simulink model "SPERTE_printer_RC"  (R2024b)
settings: Solver=FixedStepDiscrete  StartTime=0.0  StopTime=tsim  FixedStep=Ts  RelTol=1e-3  EnableMultiTasking=on
InitFcn:
  | Fs = 1000; Ts = 1/Fs;tsim = Inf;
values from neighbouring files (symbols this model uses):
  N = length(r)    [SimExpRC_SPERTE.m]
  N_RC_activate = 5    [SimExpRC_SPERTE.m]
  N_trial = 50    [SimExpRC_SPERTE.m]
  p_Q = M    (= 50)    [DesignControllerRC.m]
undefined symbols (not defined in the file or in its folder): DiscIntNeverNeededParam, p_L
libraries: simulink x7, sperte_lib x3, cstblocks x2
(part 1 of 2)
settings Model: SimulationMode=external  ExtModeTrigDuration=2  Creator=glife  LastModifiedBy=20202036
settings SolverCC: AlgebraicLoopSolver=TrustRegion  PositivePriorityOrder=on
settings DataIOCC: SaveOutput=off  DSMLogging=off  SaveTime=off  ReturnWorkspaceOutputs=off
settings OptimizationCC: EnhancedBackFolding=on  PassReuseOutputArgsThreshold=0  MaxStackSize=200000  OptimizeBlockOrder=speed  DifferentSizesBufferReuse=on  OptimizationCustomize=off
settings DebuggingCC: ParameterTunabilityLossMsg=error  UnconnectedInputMsg=warning  UnconnectedOutputMsg=warning  UnconnectedLineMsg=warning  ArithmeticOperatorsInVariantConditions=warning
settings HardwareCC: ProdBitPerLong=64  ProdLargestAtomicInteger=LongLong  ProdLargestAtomicFloat=Double  ProdLongLongMode=on  ProdHWDeviceType=ARM Compatible->ARM Cortex-A (64-bit)  UseEmbeddedCoderFeatures=off
settings ModelReferenceCC: EnableRefExpFcnMdlSchedulingChecks=on
settings SFSimCC: CustomCodeUndefinedFunction=UseInterfaceOnly
settings RTWCC: Description=Embedded Coder  SystemTargetFile=ert.tlc  HardwareBoard=Raspberry Pi (64bit)  TLCOptions="-aInlineSetEventsForThisBaseRateFcn=TLC_FALSE -aSuppressMultiTaskScheduler=TLC_FALSE  -aRateBasedStepFcn=0"  TemplateMakefile=ert_default_tmf  PostCodeGenCommand=codertarget.postCodeGenHookCommand(h); SPERTE_postGenFunc(modelName, buildInfo);  CustomSource=MW_custom_RTOS.c  CustomDefine=COREAFFINITYREQUIRED  Toolchain=GNU GCC Embedded Linux  BuildConfiguration=Faster Runs  GPUComputeCapability=3.5
settings CodeAppCC: ForceParamTrailComments=on  OperatorAnnotations=on
settings ERTTargetCC: CodeReplacementLibrary=GNU C99 extensions  ERTCustomFileBanners=off  SupportContinuousTime=on  SupportNonInlinedSFcns=on  RemoveResetFunc=off  SupportVariableSizeSignals=on  ModelStepFunctionPrototypeControlCompliant=off  ExtMode=on  ExtModeTransport=2  ExtModeStaticAlloc=on  ExtModeMexFile=ext_xcp  ExtModeMexArgs='131.155.56.35' 1 17725  ExtModeIntrfLevel=Level2 - Open  InlinedParameterPlacement=Hierarchical  ERTSrcFileBannerTemplate=codertarget_code_template.cgt  ERTHdrFileBannerTemplate=codertarget_code_template.cgt  ERTDataSrcFileTemplate=codertarget_code_template.cgt  ERTDataHdrFileTemplate=codertarget_code_template.cgt  DynamicArrayContainerType=coder::array

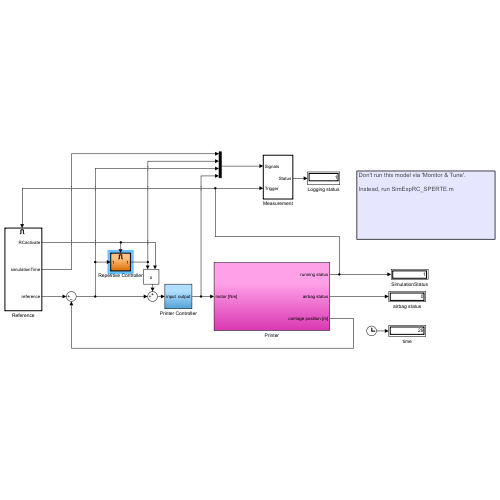
[thumbnail: Simulink's stored preview of the top-level diagram]
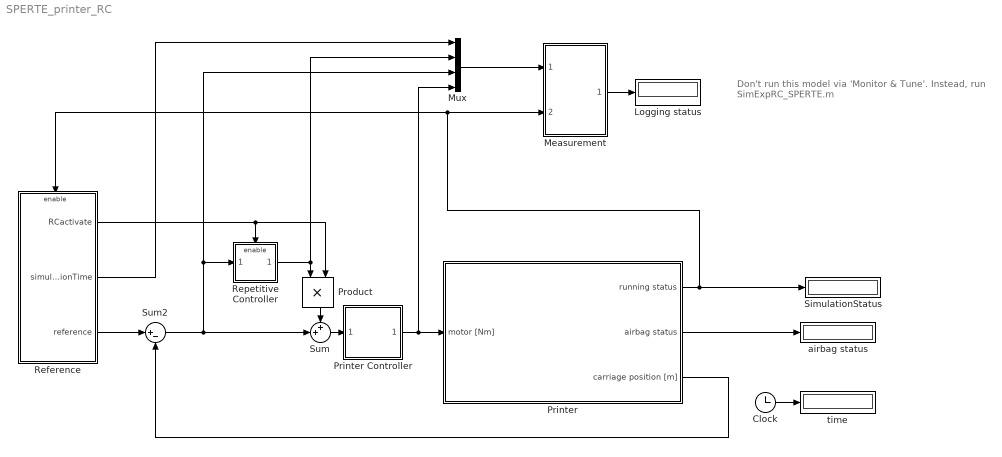
== system SPERTE_printer_RC ==
  note: Don't run this model via 'Monitor & Tune'.
      |
      | Instead, run SimExpRC_SPERTE.m
  Clock : Clock
  Logging status : Display
  Measurement : Subsystem  TreatAsAtomicUnit=on
  Mux : Mux
  Printer : Subsystem
  Printer Controller : Subsystem
  Product : Product
  Reference : Subsystem  TreatAsAtomicUnit=on
  Repetitive Controller : Subsystem  InitFcn=load('RCController.mat');
  SimulationStatus : Display
      settings: Decimation=50
  Sum : Sum  Inputs=++|
  Sum2 : Sum  Inputs=|+-
  airbag status : Display
      settings: Decimation=50
  time : Display
      settings: Decimation=50
  wires:
  Printer/3(carriage position [m]) -> Sum2/2
  Printer/2(airbag status) -> airbag status/1
  Sum2/1 -> Mux/3, Repetitive Controller/1(Input), Sum/2
  Printer Controller/1(output) -> Mux/4, Printer/1(motor [Nm])
  Clock/1 -> time/1
  Reference/3(reference) -> Sum2/1
  Mux/1 -> Measurement/1(Signals)
  Measurement/1(Status) -> Logging status/1
  Sum/1 -> Printer Controller/1(input)
  Product/1 -> Sum/1
  Repetitive Controller/1(Output) -> Mux/2, Product/1
  Reference/1(RCactivate) -> Product/2, Repetitive Controller/Enable
  Reference/2(simulationTime) -> Mux/1
  Printer/1(running status) -> Measurement/2(Trigger), Reference/Enable, SimulationStatus/1

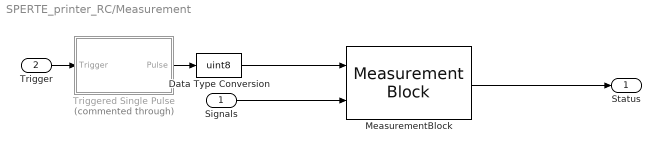
== system SPERTE_printer_RC/Measurement ==
  Signals : Inport
  Trigger : Inport  Port=2
  Data Type Conversion : DataTypeConversion  OutDataTypeStr=uint8  SaturateOnIntegerOverflow=off  RndMeth=Floor
  MeasurementBlock : sperte_lib/Measurement/Measurement Block  Description=|  Priority=-1  N_samples=N*N_trial  triggertype=0  trigger_command=1
      | Perform on-demand measurements to file using this block.
      | 
      | It can be used in 2 ways:
      | 1) Set the mask triggertype parameter to manual and use the trigger input signal to trigger a measurement.
      | You can do this by providing a 0 to 1 transition.
      | Keep it low after you start/complete the measurement, or it will measure again.
      | A file is created with measurement_0,1,2... etc
      | 
      | 2) Keep the model running, and trigger a measurement from the commandline or Matlab script.
      | For example:
      | 
      | % How many samples to measure?
      | N_samples = Fs*5;
      | % Do the measurement
      | SPERTE_Perform_Measurement(N_samples);
      | % Get the latest file
      | file_list = SPERTE_Get_Latest_Measurement(p,1,'./data');
      | % How many signals did you record?
      | N_signals = 3;
      | % Convert the .bin to .mat and return the results
      | measurement = SPERTE_Bin_To_Mat(file_list,N_signals);
      settings: SourceProductName=SPERTE library
  Triggered Single Pulse : Subsystem  Commented=through  TreatAsAtomicUnit=on  mask(single pulse generation){p_wid=20}
      mask prompts: p_wid "pulse width (number of samples)"
      mask help: This block generate a single pulse whenever a trigger happen. The pulse width must specified as a number of samples. for example if your sampling time is 0.1s and you want 3s pulse , then you should enter 30 as a pulse width.
      mask Display:
      | plot([0],[0])
      | plot([11],[0])
      | plot([5],[0.5])
      | plot([4 5 5 6 6 7],[0 0 0.25 0.25 0 0])
      | plot([5],[-0.3])
      | 
      | port_label('output', 1, 'Pulse')
      | port_label('input', 1, 'Trigger')
  Status : Outport
  wires:
  Data Type Conversion/1 -> MeasurementBlock/1
  MeasurementBlock/1 -> Status/1
  Signals/1 -> MeasurementBlock/2
  Triggered Single Pulse/1(Pulse) -> Data Type Conversion/1
  Trigger/1 -> Triggered Single Pulse/1(Trigger)

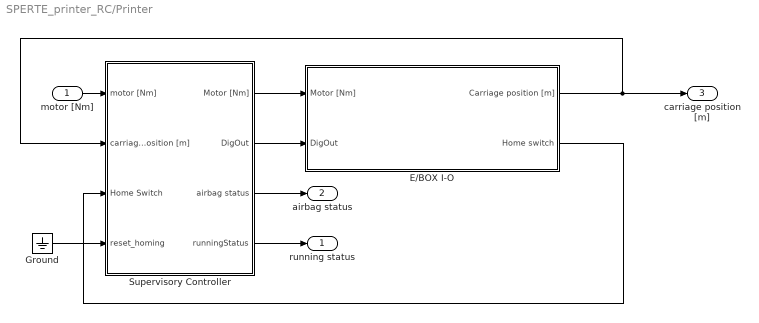
== system SPERTE_printer_RC/Printer ==
  motor [Nm] : Inport
  E/BOX I-O : Subsystem
  Ground : Ground
  Supervisory Controller : Subsystem
  running status : Outport
  airbag status : Outport  Port=2
  carriage position [m] : Outport  Port=3
  wires:
  E/BOX I-O/1(Carriage position [m]) -> Supervisory Controller/2(carriage position [m]), carriage position [m]/1
  Supervisory Controller/1(Motor [Nm]) -> E/BOX I-O/1(Motor [Nm])
  E/BOX I-O/2(Home switch) -> Supervisory Controller/3(Home Switch)
  motor [Nm]/1 -> Supervisory Controller/1(motor [Nm])
  Supervisory Controller/3(airbag status) -> airbag status/1
  Supervisory Controller/4(runningStatus) -> running status/1
  Supervisory Controller/2(DigOut) -> E/BOX I-O/2(DigOut)
  Ground/1 -> Supervisory Controller/4(reset_homing)

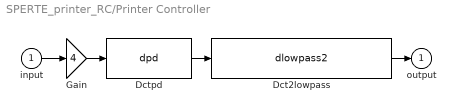
== system SPERTE_printer_RC/Printer Controller ==
  input : Inport
  Dct2lowpass : S-Function  FunctionName=dlowpass2  Parameters=f_den, b_den, 0.001  SFunctionDeploymentMode=off  EnableBusSupport=off  mask(dctools){f_den=40, b_den=0.7}
      mask prompts: f_den "Pole [Hz]"; b_den "Damping pole [-]"
      mask help: This block implements a discrete time 2nd order lowpass filter.
      mask Display: disp('DCT 2nd order lowpass')
  Dctpd : S-Function  FunctionName=dpd  Parameters=kp, kv, 0.001  SFunctionDeploymentMode=off  EnableBusSupport=off  mask(dctools){kp=40, kv=1}
      mask help: This block implements a discrete time pd filter.
      mask Display: disp('DCT pd')
  Gain : Gain  Gain=4  SaturateOnIntegerOverflow=on  OutDataTypeStr=Inherit: Same as input  ParamDataTypeStr=Inherit: Same as input
  output : Outport
  wires:
  input/1 -> Gain/1
  Gain/1 -> Dctpd/1
  Dctpd/1 -> Dct2lowpass/1
  Dct2lowpass/1 -> output/1

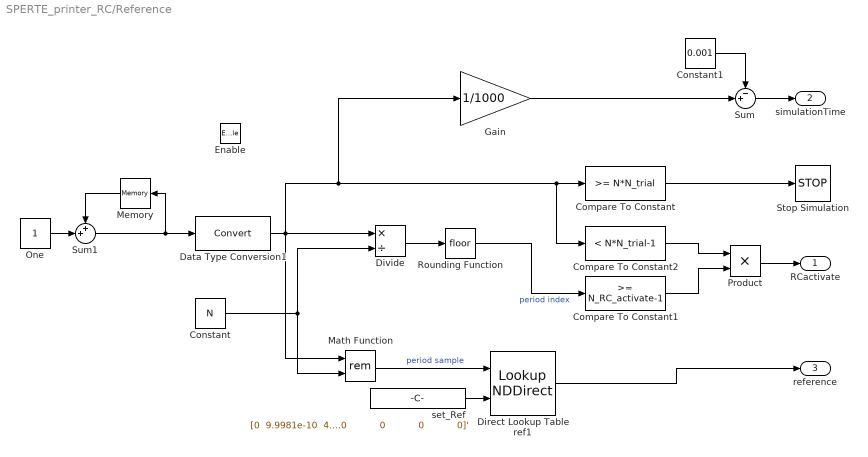
== system SPERTE_printer_RC/Reference ==
  Enable : EnablePort  StatesWhenEnabling=reset
  Compare To Constant : simulink/Logic and Bit Operations/Compare To Constant  relop=>=  const=N*N_trial  OutDataTypeStr=boolean
  Compare To Constant1 : simulink/Logic and Bit Operations/Compare To Constant  relop=>=  const=N_RC_activate-1  OutDataTypeStr=boolean
  Compare To Constant2 : simulink/Logic and Bit Operations/Compare To Constant  relop=<  const=N*N_trial-1  OutDataTypeStr=boolean
  Constant : Constant  Value=N
  Constant1 : Constant  Value=0.001
  Data Type Conversion1 : DataTypeConversion  SaturateOnIntegerOverflow=off  RndMeth=Floor
  Direct Lookup Table ref1 : LookupNDDirect  NumberOfTableDimensions=1  TableIsInput=on  Table=[4 5 ;16 19 ]  DiagnosticForOutOfRangeInput=Error
  Divide : Product  Inputs=*/
  Gain : Gain  Gain=1/1000
  Math Function : Math  Operator=rem  SignedPower=on
  Memory : Memory
  One : Constant  OutDataTypeStr=Inherit: Inherit via back propagation
  Product : Product
  Rounding Function : Rounding
  Stop Simulation : Stop
  Sum : Sum  Inputs=-+|
  Sum1 : Sum  Inputs=++|
  set_Ref : Constant  Value="[0  9.9981e-10  4.9991e-09  1.4997e-08  3.4993e-08  6.9987e-08  1.2598e-07  2.0996e-07  3.2994e-07  4.9491e-07  7.1487e-07  1.0008e-06  1.3647e-06  1.8197e-06  2.3796e-06  3.0594e-06  3.8753e-06  4.8441e-06  5.9839e-06  7.3136e-06  8.8533e-06  1.0624e-05  1.2648e-05  1.4947e-05  1.7547e-05  2.0471e-05  2.3747e-05    2.74e-05  3.1459e-05  3.5953e-05  4.0912e-05  4.6367e-05   5.235e-05  5.8894e-05  6.6033e-05  7.3801e-05  8.2236e-05  9.1373e-05  0.00010125  0.00011191  0.00012339  0.00013573  0.00014897  0.00016315  0.00017833  0.00019454  0.00021184  0.00023026  0.00024985  0.00027067  0.00029277  0.00031619  0.00034099  0.00036722  0.00039494  0.00042419  0.00045504  0.00048754  0.00052176  0.00055774  0.00059555  0.00063526  0.00067691  0.00072058  0.00076633  0.00081422  0.00086431  0.00091665  0.00097131   0.0010283   0.0010878   0.0011497   0.0012142   0.0012813    0.001351   0.0014234   0.0014986   0.0015765   0.0016573    0.001741   0.0018276   0.0019172   0.0020098   0.0021054   0.0022042   0.0023062   0.0024113   0.0025196   0.0026312   0.0027461   0.0028644    0.002986    0.003111   0.0032395   0.0033715   0.0035069   0.0036459   0.0037884   0.0039346   0.0040843   0.0042377   0.0043948   0.0045555     0.00472   0.0048882   0.0050602   0.0052359   0.0054154   0.0055988    0.005786    0.005977   0.0061719   0.0063707   0.0065734   0.0067799   0.0069904   0.0072048   0.0074232   0.0076454   0.0078717   0.0081018    0.008336   0.0085741   0.0088161   0.0090622   0.0093122   0.0095661   0.0098241    0.010086    0.010352    0.010622    0.010895    0.011173    0.011455     0.01174     0.01203    0.012323    0.012621    0.012922    0.013227    0.013536    0.013849    0.014165    0.014486     0.01481    0.015138     0.01547    0.015806    0.016145    0.016488    0.016834    0.017185    0.017538    0.017896    0.018257    0.018621     0.01899    0.019361    0.019736    0.020114    0.020496    0.020881     0.02127    0.021661    0.022056    0.022454    0.022855     0.02326    0.023667    0.024078    0.024491    0.024907    0.025327    0.025749    0.026173    0.026601    0.027031    0.027464      0.0279    0.028338    0.028778    0.029221    0.029667    0.030114    0.030564    0.031016    0.031471    0.031927    0.032385    0.032846    0.033308    0.033772    0.034238    0.034705    0.035174    0.035645    0.036117    0.036591    0.037066    0.037543    0.038021      0.0385     0.03898    0.039462    0.039945    0.040428    0.040913    0.041399    0.041886    0.042373    0.042862    0.043351    0.043841    0.044332    0.044824    0.045316    0.045809    0.046302    0.046796    0.047291    0.047786    0.048281    0.048777    0.049274     0.04977    0.050268    0.050765    0.051263    0.051761    0.052259    0.052757    0.053256    0.053755    0.054254    0.054753    0.055252    0.055752    0.056251    0.056751    0.057251     0.05775     0.05825     0.05875     0.05925     0.05975     0.06025     0.06075     0.06125     0.06175     0.06225     0.06275     0.06325     0.06375     0.06425     0.06475     0.06525     0.06575     0.06625     0.06675     0.06725     0.06775     0.06825     0.06875     0.06925     0.06975     0.07025     0.07075     0.07125     0.07175     0.07225     0.07275     0.07325     0.07375     0.07425     0.07475     0.07525     0.07575     0.07625     0.07675     0.07725     0.07775     0.07825     0.07875     0.07925     0.07975     0.08025     0.08075     0.08125     0.08175     0.08225     0.08275     0.08325     0.08375     0.08425     0.08475     0.08525     0.08575     0.08625     0.08675     0.08725     0.08775     0.08825     0.08875     0.08925     0.08975     0.09025     0.09075     0.09125     0.09175     0.09225     0.09275     0.09325     0.09375     0.09425     0.09475     0.09525     0.09575     0.09625     0.09675     0.09725     0.09775     0.09825     0.09875     0.09925     0.09975     0.10025     0.10075     0.10125     0.10175     0.10225     0.10275     0.10325     0.10375     0.10425 ...(+17687 chars)]'"
  RCactivate : Outport  InitialOutput=0
  simulationTime : Outport  Port=2  InitialOutput=0
  reference : Outport  Port=3  InitialOutput=0
  wires:
  Divide/1 -> Rounding Function/1
  Rounding Function/1 -> Compare To Constant1/1  "period index"
  Compare To Constant2/1 -> Product/1
  Data Type Conversion1/1 -> Divide/1, Gain/1, Compare To Constant2/1, Compare To Constant/1, Math Function/1
  Compare To Constant/1 -> Stop Simulation/1
  Direct Lookup Table ref1/1 -> reference/1
  Gain/1 -> Sum/2
  Constant/1 -> Divide/2, Math Function/2
  Product/1 -> RCactivate/1
  Sum1/1 -> Data Type Conversion1/1, Memory/1
  Compare To Constant1/1 -> Product/2
  Math Function/1 -> Direct Lookup Table ref1/1  "period sample"
  set_Ref/1 -> Direct Lookup Table ref1/2
  Memory/1 -> Sum1/1
  One/1 -> Sum1/2
  Sum/1 -> simulationTime/1
  Constant1/1 -> Sum/1

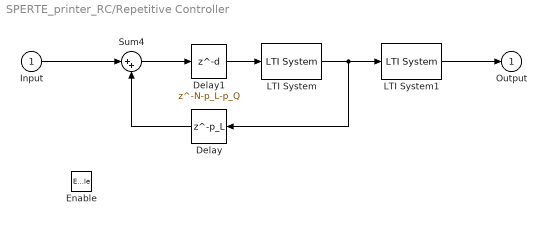
== system SPERTE_printer_RC/Repetitive Controller ==
  Input : Inport
  Enable : EnablePort  StatesWhenEnabling=reset
  Delay : Delay  DelayLength=p_L  InitialCondition=0
  Delay1 : Delay  DelayLength=N-p_L-p_Q  InitialCondition=0
  LTI System : cstblocks/LTI System  sys=Q_c  IC=[]  PadeOrder=0
  LTI System1 : cstblocks/LTI System  sys=L_c  IC=[]  PadeOrder=0
  Sum4 : Sum  Inputs=|++  InputSameDT=on  SaturateOnIntegerOverflow=on  OutDataTypeStr=Inherit: Same as first input
  Output : Outport  InitialOutput=[0]
  wires:
  Input/1 -> Sum4/1
  LTI System1/1 -> Output/1
  Sum4/1 -> Delay1/1
  Delay/1 -> Sum4/2
  Delay1/1 -> LTI System/1
  LTI System/1 -> LTI System1/1, Delay/1

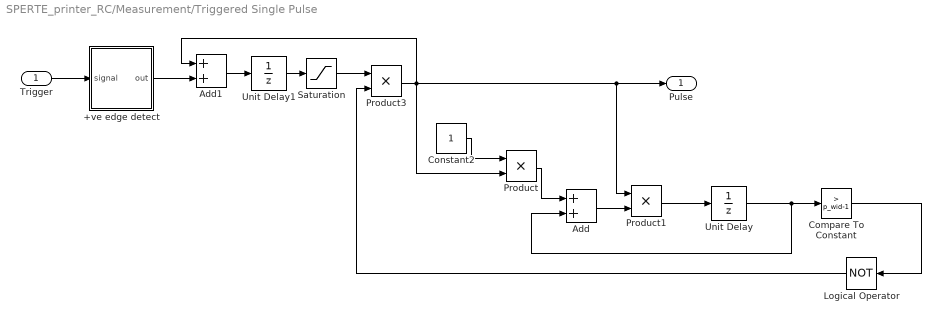
== system SPERTE_printer_RC/Measurement/Triggered Single Pulse ==
  Trigger : Inport
  +ve edge detect : Subsystem
  Add : Sum
  Add1 : Sum
  Compare To Constant : simulink/Logic and Bit Operations/Compare To Constant  relop=>  const=p_wid-1  OutDataTypeStr=boolean
  Constant2 : Constant
  Logical Operator : Logic  Operator=NOT  AllPortsSameDT=off  OutDataTypeStr=boolean
  Product : Product  RndMeth=Zero
  Product1 : Product  RndMeth=Zero
  Product3 : Product  RndMeth=Zero
  Saturation : Saturate  UpperLimit=1  LowerLimit=0
  Unit Delay : UnitDelay  SampleTime=-1  HasFrameUpgradeWarning=on
  Unit Delay1 : UnitDelay  SampleTime=-1  HasFrameUpgradeWarning=on
  Pulse : Outport
  wires:
  Compare To Constant/1 -> Logical Operator/1
  Constant2/1 -> Product/1
  Product/1 -> Add/1
  Unit Delay/1 -> Add/2, Compare To Constant/1
  Trigger/1 -> +ve edge detect/1(signal)
  +ve edge detect/1(out) -> Add1/2
  Add/1 -> Product1/2
  Product1/1 -> Unit Delay/1
  Add1/1 -> Unit Delay1/1
  Unit Delay1/1 -> Saturation/1
  Saturation/1 -> Product3/1
  Product3/1 -> Add1/1, Product/2, Product1/1, Pulse/1
  Logical Operator/1 -> Product3/2

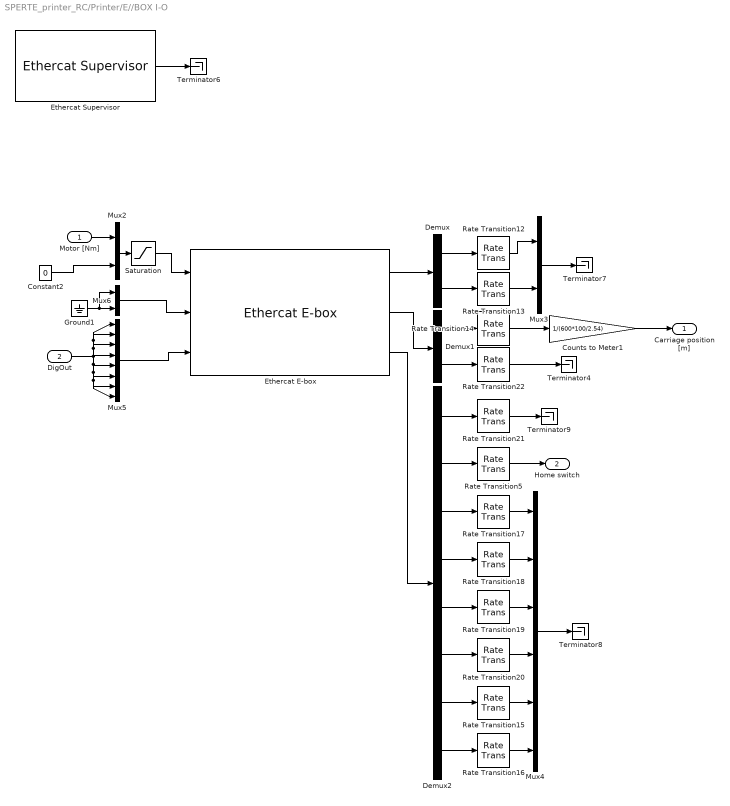
== system SPERTE_printer_RC/Printer/E//BOX I-O ==
  Motor [Nm] : Inport
  DigOut : Inport  Port=2
  Constant2 : Constant  Value=0
  Counts to Meter1 : Gain  Gain=1/(600*100/2.54)
  Demux : Demux  Outputs=2
  Demux1 : Demux  Outputs=2
  Demux2 : Demux  Outputs=8
  Ethercat E-box : sperte_lib/EtherCAT/Ethercat E-box  Priority=-2  link_id=0
      settings: SourceProductName=SPERTE library
  Ethercat Supervisor : sperte_lib/EtherCAT/Ethercat Supervisor  Description=Must be executed first, keep at -1 priority (highest)  Priority=-3  portid=0  ectimeout=500
      settings: SourceProductName=SPERTE library
  Ground1 : Ground
  Mux2 : Mux  Inputs=2
  Mux3 : Mux  Inputs=2
  Mux4 : Mux  Inputs=6
  Mux5 : Mux  Inputs=8
  Mux6 : Mux  Inputs=2
  Rate Transition{5,12..22} (12 alike) : RateTransition
  Saturation : Saturate  UpperLimit=2.5  LowerLimit=-2.5
  Terminator{4,6..9} (5 alike) : Terminator
  Carriage position [m] : Outport
  Home switch : Outport  Port=2
  wires:
  Motor [Nm]/1 -> Mux2/1
  Demux2/2 -> Rate Transition5/1
  Rate Transition5/1 -> Home switch/1
  Saturation/1 -> Ethercat E-box/1
  Ethercat E-box/3 -> Demux2/1
  Ground1/1 -> Mux6/1, Mux6/2
  Ethercat Supervisor/1 -> Terminator6/1
  Ethercat E-box/2 -> Demux1/1
  Constant2/1 -> Mux2/2
  Mux2/1 -> Saturation/1
  Counts to Meter1/1 -> Carriage position [m]/1
  Ethercat E-box/1 -> Demux/1
  Demux/1 -> Rate Transition12/1
  Demux/2 -> Rate Transition13/1
  Rate Transition13/1 -> Mux3/2
  Mux3/1 -> Terminator7/1
  Rate Transition12/1 -> Mux3/1
  Rate Transition14/1 -> Counts to Meter1/1
  Demux1/1 -> Rate Transition14/1
  Demux1/2 -> Rate Transition22/1
  Rate Transition19/1 -> Mux4/3
  Rate Transition18/1 -> Mux4/2
  Rate Transition20/1 -> Mux4/4
  Demux2/8 -> Rate Transition16/1
  Rate Transition17/1 -> Mux4/1
  Demux2/5 -> Rate Transition19/1
  Demux2/6 -> Rate Transition20/1
  Demux2/4 -> Rate Transition18/1
  Rate Transition15/1 -> Mux4/5
  Mux4/1 -> Terminator8/1
  Demux2/3 -> Rate Transition17/1
  Demux2/7 -> Rate Transition15/1
  Rate Transition16/1 -> Mux4/6
  Rate Transition21/1 -> Terminator9/1
  Demux2/1 -> Rate Transition21/1
  Mux5/1 -> Ethercat E-box/3
  DigOut/1 -> Mux5/8, Mux5/7, Mux5/6, Mux5/5, Mux5/4, Mux5/1, Mux5/2, Mux5/3
  Mux6/1 -> Ethercat E-box/2
  Rate Transition22/1 -> Terminator4/1

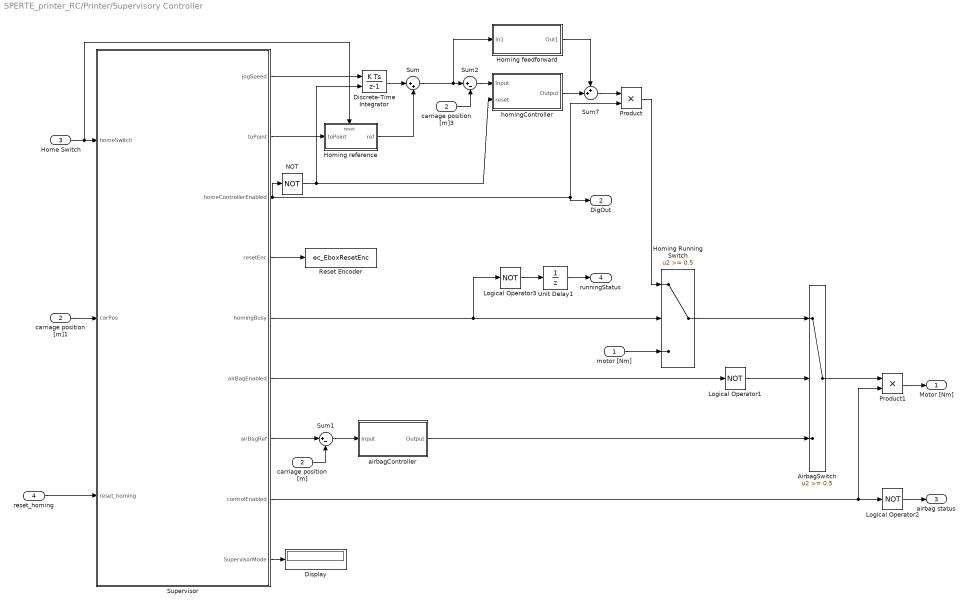
== system SPERTE_printer_RC/Printer/Supervisory Controller ==
  motor [Nm] : Inport
  carriage position [m] : Inport  Port=2
  Home Switch : Inport  Port=3
  reset_homing : Inport  Port=4
  AirbagSwitch : Switch  Threshold=0.5  SaturateOnIntegerOverflow=off  InputSameDT=off
  Discrete-Time Integrator : DiscreteIntegrator  ExternalReset=level  SampleTime=-1  ICPrevOutput=DiscIntNeverNeededParam  ICPrevScaledInput=DiscIntNeverNeededParam
  Display : Display
  Homing Running Switch : Switch  Threshold=0.5  SaturateOnIntegerOverflow=off  InputSameDT=off
  Homing feedforward : Subsystem
  Homing reference : Subsystem
  Logical Operator1 : Logic  Operator=NOT  AllPortsSameDT=off  OutDataTypeStr=boolean
  Logical Operator2 : Logic  Operator=NOT  AllPortsSameDT=off  OutDataTypeStr=boolean
  Logical Operator3 : Logic  Operator=NOT  AllPortsSameDT=off  OutDataTypeStr=boolean
  NOT : Logic  Operator=NOT  IconShape=distinctive  AllPortsSameDT=off  OutDataTypeStr=boolean
  Product : Product  RndMeth=Zero
  Product1 : Product  RndMeth=Zero
  Reset Encoder : S-Function  FunctionName=ec_EboxResetEnc  Parameters=link_id  SFunctionDeploymentMode=off  EnableBusSupport=off  mask{link_id=0}
      mask prompts: link_id "analog in id (start from 1)"
  Sum : Sum  Inputs=|++
  Sum1 : Sum  Inputs=|+-
  Sum2 : Sum  Inputs=|+-
  Sum7 : Sum  Inputs=++|
  Supervisor : Stateflow chart  TreatAsAtomicUnit=on
  Unit Delay1 : UnitDelay  SampleTime=-1  HasFrameUpgradeWarning=on
  airbagController : Subsystem
  carriage position [m]1 : InportShadow  Port=2
  carriage position [m]3 : InportShadow  Port=2
  homingController : Subsystem
  Motor [Nm] : Outport
  DigOut : Outport  Port=2
  airbag status : Outport  Port=3
  runningStatus : Outport  Port=4
  wires:
  Homing Running Switch/1 -> AirbagSwitch/1
  Sum/1 -> Homing feedforward/1(In1), Sum2/1
  Sum2/1 -> homingController/1(Input)
  Home Switch/1 -> Homing reference/Reset, Supervisor/1(homeSwitch)
  Supervisor/1(jogSpeed) -> Discrete-Time Integrator/1
  carriage position [m]3/1 -> Sum2/2
  motor [Nm]/1 -> Homing Running Switch/3
  homingController/1(Output) -> Sum7/2
  Product/1 -> Homing Running Switch/1
  Discrete-Time Integrator/1 -> Sum/1
  Supervisor/5(homingBusy) -> Homing Running Switch/2, Logical Operator3/1
  Supervisor/3(homeControllerEnabled) -> Product/2, DigOut/1, NOT/1
  Supervisor/2(toPoint) -> Homing reference/1(toPoint)
  Supervisor/4(resetEnc) -> Reset Encoder/1
  carriage position [m]1/1 -> Supervisor/2(carPos)
  Supervisor/6(airBagEnabled) -> Logical Operator1/1
  Logical Operator1/1 -> AirbagSwitch/2
  airbagController/1(Output) -> AirbagSwitch/3
  Sum1/1 -> airbagController/1(Input)
  carriage position [m]/1 -> Sum1/2
  Supervisor/7(airBagRef) -> Sum1/1
  AirbagSwitch/1 -> Product1/1
  Product1/1 -> Motor [Nm]/1
  Supervisor/8(controlEnabled) -> Logical Operator2/1, Product1/2
  Logical Operator2/1 -> airbag status/1
  Logical Operator3/1 -> Unit Delay1/1
  Supervisor/9(SupervisorMode) -> Display/1
  Unit Delay1/1 -> runningStatus/1
  reset_homing/1 -> Supervisor/3(reset_homing)
  NOT/1 -> homingController/2(reset), Discrete-Time Integrator/2
  Sum7/1 -> Product/1
  Homing reference/1(ref) -> Sum/2
  Homing feedforward/1(Out1) -> Sum7/1

== system SPERTE_printer_RC/Measurement/Triggered Single Pulse/+ve edge detect ==
  note: Edge
  signal : Inport
  Delay Input1 : UnitDelay  Description=Store in Global RAM  DisableCoverage=on  SampleTime=-1  HasFrameUpgradeWarning=on
  FixPt Relational Operator : RelationalOperator  Operator=>  OutDataTypeStr=fixdt(0, 8)  ZeroCross=off  InputSameDT=off
  Positive : simulink/Logic and Bit Operations/Compare To Zero  relop=>  OutDataTypeStr=uint8  ZeroCross=off
  out : Outport
  wires:
  Delay Input1/1 -> FixPt Relational Operator/2  "U(k-1)"
  Positive/1 -> Delay Input1/1, FixPt Relational Operator/1  "U(k)"
  FixPt Relational Operator/1 -> out/1
  signal/1 -> Positive/1

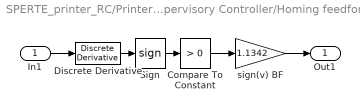
== system SPERTE_printer_RC/Printer/Supervisory Controller/Homing feedforward ==
  In1 : Inport
  Compare To Constant : simulink/Logic and Bit Operations/Compare To Constant  relop=>  const=0  OutDataTypeStr=uint8
  Discrete Derivative : simulink/Discrete/Discrete Derivative  gainval=1.0  ICPrevScaledInput=0.0  OutMin=[]  OutMax=[]  OutDataType=fixdt(1, 16)  OutScaling=2^-10  DoSatur=off
  Sign : Signum
  sign(v) BF : Gain  Gain=1.1342
  Out1 : Outport
  wires:
  In1/1 -> Discrete Derivative/1
  Discrete Derivative/1 -> Sign/1
  Sign/1 -> Compare To Constant/1
  Compare To Constant/1 -> sign(v) BF/1
  sign(v) BF/1 -> Out1/1

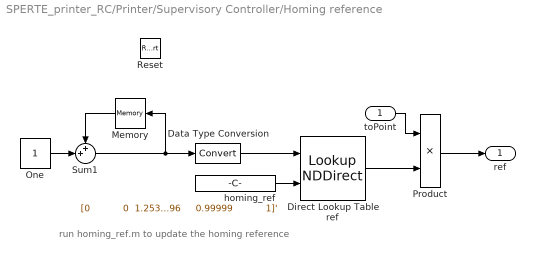
== system SPERTE_printer_RC/Printer/Supervisory Controller/Homing reference ==
  note: run homing_ref.m to update the homing reference
  toPoint : Inport
  Reset : ResetPort  DisableCoverage=on
  Data Type Conversion : DataTypeConversion  SaturateOnIntegerOverflow=off  RndMeth=Floor
  Direct Lookup Table ref : LookupNDDirect  NumberOfTableDimensions=1  TableIsInput=on  Table=[4 5 ;16 19 ]  DiagnosticForOutOfRangeInput=Error
  Memory : Memory
  One : Constant  OutDataTypeStr=Inherit: Inherit via back propagation
  Product : Product  OutDataTypeStr=double
  Sum1 : Sum  Inputs=++|
  homing_ref : Constant  Value="[0           0  1.2531e-05  3.7594e-05  7.5188e-05  0.00012531  0.00018797  0.00026316  0.00035088  0.00045113  0.00056391  0.00068922  0.00082707  0.00097744   0.0011404   0.0013158   0.0015038   0.0017043   0.0019173   0.0021429    0.002381   0.0026316   0.0028947   0.0031704   0.0034586   0.0037594   0.0040727   0.0043985   0.0047368   0.0050877   0.0054511   0.0058271   0.0062155   0.0066165   0.0070301   0.0074561   0.0078947   0.0083459   0.0088095   0.0092857   0.0097744    0.010276    0.010789    0.011316    0.011855    0.012406     0.01297    0.013546    0.014135    0.014737    0.015351    0.015977    0.016617    0.017268    0.017932    0.018609    0.019298        0.02    0.020714    0.021441     0.02218    0.022932    0.023697    0.024474    0.025263    0.026065     0.02688    0.027707    0.028546    0.029398    0.030263     0.03114     0.03203    0.032932    0.033847    0.034774    0.035714    0.036667    0.037632    0.038609    0.039599    0.040602    0.041617    0.042644    0.043684    0.044737    0.045802     0.04688     0.04797    0.049073    0.050188    0.051316    0.052456    0.053609    0.054774    0.055952    0.057143    0.058346    0.059561    0.060789     0.06203    0.063283    0.064549    0.065827    0.067118    0.068421    0.069737    0.071065    0.072406    0.073759    0.075125    0.076504    0.077895    0.079298    0.080714    0.082143    0.083584    0.085038    0.086504    0.087982    0.089474    0.090977    0.092494    0.094023    0.095564    0.097118    0.098684     0.10026     0.10185     0.10346     0.10508      0.1067     0.10835        0.11     0.11167     0.11335     0.11504     0.11674     0.11846     0.12019     0.12193     0.12368     0.12545     0.12723     0.12902     0.13083     0.13264     0.13447     0.13632     0.13817     0.14004     0.14192     0.14381     0.14571     0.14763     0.14956      0.1515     0.15346     0.15543     0.15741      0.1594      0.1614     0.16342     0.16545     0.16749     0.16955     0.17162      0.1737     0.17579     0.17789     0.18001     0.18214     0.18429     0.18644     0.18861     0.19079     0.19298     0.19519     0.19741     0.19964     0.20188     0.20414      0.2064     0.20868     0.21098     0.21328      0.2156     0.21793     0.22028     0.22263       0.225     0.22738     0.22977     0.23218      0.2346     0.23703     0.23947     0.24193      0.2444     0.24688     0.24937     0.25188     0.25439     0.25689      0.2594      0.2619     0.26441     0.26692     0.26942     0.27193     0.27444     0.27694     0.27945     0.28195     0.28446     0.28697     0.28947     0.29198     0.29449     0.29699      0.2995     0.30201     0.30451     0.30702     0.30952     0.31203     0.31454     0.31704     0.31955     0.32206     0.32456     0.32707     0.32957     0.33208     0.33459     0.33709      0.3396     0.34211     0.34461     0.34712     0.34962     0.35213     0.35464     0.35714     0.35965     0.36216     0.36466     0.36717     0.36967     0.37218     0.37469     0.37719      0.3797     0.38221     0.38471     0.38722     0.38972     0.39223     0.39474     0.39724     0.39975     0.40226     0.40476     0.40727     0.40977     0.41228     0.41479     0.41729      0.4198     0.42231     0.42481     0.42732     0.42982     0.43233     0.43484     0.43734     0.43985     0.44236     0.44486     0.44737     0.44987     0.45238     0.45489     0.45739      0.4599     0.46241     0.46491     0.46742     0.46992     0.47243     0.47494     0.47744     0.47995     0.48246     0.48496     0.48747     0.48997     0.49248     0.49499     0.49749         0.5     0.50251     0.50501     0.50752     0.51003     0.51253     0.51504     0.51754     0.52005     0.52256     0.52506     0.52757     0.53008     0.53258     0.53509     0.53759      0.5401     0.54261     0.54511     0.54762     0.55013     0.55263     0.55514     0.55764     0.56015     0.56266     0.56516     0.56767     0.57018     0.57268     0.57519     0.57769      0.5802     0.58271 ...(+3191 chars)]'"
  ref : Outport
  wires:
  toPoint/1 -> Product/1
  Direct Lookup Table ref/1 -> Product/2
  Product/1 -> ref/1
  homing_ref/1 -> Direct Lookup Table ref/2
  Memory/1 -> Sum1/1
  One/1 -> Sum1/2
  Data Type Conversion/1 -> Direct Lookup Table ref/1
  Sum1/1 -> Data Type Conversion/1, Memory/1

== system SPERTE_printer_RC/Printer/Supervisory Controller/airbagController ==
  Input : Inport
  Dct2lowpass3 : S-Function  FunctionName=dlowpass2  Parameters=f_den, b_den, 0.001  SFunctionDeploymentMode=off  EnableBusSupport=off  mask(dctools){f_den=40, b_den=0.7}
      mask prompts: f_den "Pole [Hz]"; b_den "Damping pole [-]"
      mask help: This block implements a discrete time 2nd order lowpass filter.
      mask Display: disp('DCT 2nd order lowpass')
  Dctpd2 : S-Function  FunctionName=dpd  Parameters=kp, kv, 0.001  SFunctionDeploymentMode=off  EnableBusSupport=off  mask(dctools){kp=40, kv=1}
      mask help: This block implements a discrete time pd filter.
      mask Display: disp('DCT pd')
  Gain1 : Gain  Gain=4  SaturateOnIntegerOverflow=on  OutDataTypeStr=Inherit: Same as input  ParamDataTypeStr=Inherit: Same as input
  Output : Outport
  wires:
  Input/1 -> Gain1/1
  Gain1/1 -> Dctpd2/1
  Dctpd2/1 -> Dct2lowpass3/1
  Dct2lowpass3/1 -> Output/1
